simulink model "Bruening_4t_showshuffle"  (R2015a)
settings: Solver=ode4  SolverMode=MultiTasking  StartTime=0.0  StopTime=inf  FixedStep=BKIN_STEP_TIME  RelTol=1e-3
StartFcn:
  |  warndlg('Dexterit-E models cannot run under simulation. Please compile your model and run it from within Dexterit-E.');set_param(bdroot,'SimulationCommand','stop')
model workspace (MAT data in the model file):
  BKIN_STEP_TIME = 0.00025
  col_x = 1
  col_y = 2
  E_TARGET_ON = 3
  E_HOLD_AT_TARGET = 5
  LOGICAL_RADIUS = 4
  START_TARGET_COL = 1
  END_TARGET_COL = 2
  ROTATION_CENTER = 5
  WAIT_AT_1stTARGET_COL = 7
  MAXREACHTIME_COL = 8
  DELAY_POSTTRIAL_COL = 9
  E_STAY_CENTER = 2
  VISUAL_RADIUS = 3
  COLOR = 5
  ALTCOLOR = 6
  STROKECOLOUR = 7
  STROKEWIDTH = 9
  TARGET_EGG = 6
  LABEL_TEXT = 12
  LABEL_COLOUR = 13
  LABEL_HEIGHT = 14
  TEXT_DISPLAY_TARGET = 10
  ALTSTROKECOLOUR = 8
  SEGMENT_COUNT = 11
  E_TARGET_MISS = 6
  END_X = 10
  END_Y = 11
  E_LEFT_RING = 4
  E_START_BLOCK = 10
  BKIN_KINEMATIC_FRAME_SIZE = 400
  E_NO_EVENT = 1
  TARGET_IN_USE = 3
  R_PROB = 4
  E_R_TARG1 = 7
  E_M_TARG1 = 12
  E_R_TARG2 = 8
  E_M_TARG2 = 13
  E_R_TARG3 = 9
  E_M_TARG3 = 14
  E_R_TARG4 = 11
  E_M_TARG4 = 15
  WAIT_TIME = 12
  TONE_DURATION = 13
  FLASH_INTER = 14
  FLASH_NUM = 15
  BREAK_T1 = 16
  BREAK_T2 = 17
  ALTVISUAL_RADIUS = 15
  ALTCOLOR2 = 16
undefined symbols (not defined in the file or in its folder): slselsubs
libraries: Video x15, simulink x12, xpcrtudplib x12, xpcutilitieslib x10, xpcobsoletelib x8, ethercat x2, General x2, slrtlib x2, KINARM_general x1
(part 6 of 6)

== matlab function Bruening_4t_showshuffle/DataLogging/Poll KINARM/make KINData bus/splitKINData arm1 ==
  data: robot_row input; link_lengths output; pointer_offset output; shoulder_loc output; arm_orientation output; shoulder_ang output; elbow_ang output; shoulder_velocity output; elbow_velocity output; shoulder_acceleration output; elbow_acceleration output; joint_torque_cmd output; motor_torque_cmd output; link_angle output; link_velocity output; link_acceleration output; hand_position output; hand_velocity output; hand_acceleration output; motor_status output; force_sensor_force_uvw output; force_sensor_torque_uvw output; force_sensor_force_xyz output; force_sensor_torque_xyz output; force_sensor_timestamp output
function [link_lengths, pointer_offset, shoulder_loc, arm_orientation, ...
    shoulder_ang, elbow_ang, shoulder_velocity, elbow_velocity, shoulder_acceleration, elbow_acceleration, ...
    joint_torque_cmd, motor_torque_cmd, ...
    link_angle, link_velocity, link_acceleration, ...
    hand_position, hand_velocity, hand_acceleration, ...
    motor_status, ...
    force_sensor_force_uvw, force_sensor_torque_uvw, force_sensor_force_xyz, force_sensor_torque_xyz, force_sensor_timestamp] = splitKINData(robot_row)

link_lengths = robot_row(1,1:2);                % L1, L2 length in m
pointer_offset = robot_row(1,3);                % perpendicular distance from L2 to subject pointer (m)
shoulder_loc = robot_row(1,4:5);                % shoulder x,y position (m) (global coordinates)
arm_orientation = robot_row(1,6);                % subject's expected arm orientation (1: right, 2: left)
shoulder_ang = robot_row(1,7);				% shoulder joint angle, with correction for offsets (see above) (rad)
elbow_ang = robot_row(1,8);					% elbow joint angle, with correction for offsets (see above) (rad)
shoulder_velocity = robot_row(1,9);             % shoulder joint angular velocity (rad/s)
elbow_velocity = robot_row(1,10);               % elbow joint angular velocity (rad/s)
shoulder_acceleration = robot_row(1,11);        % shoulder joint angular acceleration (rad/s^2)
elbow_acceleration = robot_row(1,12);           % elbow joint angular acceleration (rad/s^2)
joint_torque_cmd = robot_row(1,13:14);          % commanded shoulder (1), and elbow (2) torque (Nm)
motor_torque_cmd = robot_row(1,15:16);          % commanded motor 1 (1) and 2 (2) torque (shoulder torque less elbow torque) (Nm)

link_angle = robot_row(1,17:18);                % upper arm angle with corrections, orientation-independent (see above) (rad)
link_velocity = robot_row(1,19:20);             % upper arm angular velocity, orientation-independent (see above) (rad/s)
link_acceleration = robot_row(1,21:22);         % upper arm angular acceleration, orientation-independent (see above) (rad/s^2)


hand_position = robot_row(1,23:24);             % fingertip position in x,y (m)
hand_velocity = robot_row(1,25:26);             % fingertip velocity in x,y (m/s)
hand_acceleration = robot_row(1,27:28);         % fingertip acceleration in x,y (m/s^2)

% shoulder_velocity_filt = robot_row(1,35);
% elbow_velocity_filt = robot_row(1,36);

motor_status = robot_row(1,37);                 % motor status (bitfield; each 0: motor enabled, 1: motor disabled/faulted)

force_sensor_force_uvw = robot_row(1,38:40);    % force measured by force sensor along u,v,w in its local coordinate system (N)
force_sensor_torque_uvw = robot_row(1,41:43);   % torque measured by force sensor along u,v,w in its local coordinate system (Nm)

force_sensor_force_xyz = robot_row(1,44:46);    % force measured by force sensor along x,y,z in the global coordinate system (N)
force_sensor_torque_xyz = robot_row(1,47:49);   % torque measured by force sensor along x in its local coordinate system (Nm)
force_sensor_timestamp = robot_row(1,50);       % The timestamp from the force sensor(s)

end

== matlab function Bruening_4t_showshuffle/DataLogging/Poll KINARM/make KINData bus/splitKINData arm2 ==
  data: robot_row input; link_lengths output; pointer_offset output; shoulder_loc output; arm_orientation output; shoulder_ang output; elbow_ang output; shoulder_velocity output; elbow_velocity output; shoulder_acceleration output; elbow_acceleration output; joint_torque_cmd output; motor_torque_cmd output; link_angle output; link_velocity output; link_acceleration output; hand_position output; hand_velocity output; hand_acceleration output; motor_status output; force_sensor_force_uvw output; force_sensor_torque_uvw output; force_sensor_force_xyz output; force_sensor_torque_xyz output; force_sensor_timestamp output
function [link_lengths, pointer_offset, shoulder_loc, arm_orientation, ...
    shoulder_ang, elbow_ang, shoulder_velocity, elbow_velocity, shoulder_acceleration, elbow_acceleration, ...
    joint_torque_cmd, motor_torque_cmd, ...
    link_angle, link_velocity, link_acceleration, ...
    hand_position, hand_velocity, hand_acceleration, ...
    motor_status, ...
    force_sensor_force_uvw, force_sensor_torque_uvw, force_sensor_force_xyz, force_sensor_torque_xyz, force_sensor_timestamp] = splitKINData(robot_row)

link_lengths = robot_row(1,1:2);                % L1, L2 length in m
pointer_offset = robot_row(1,3);                % perpendicular distance from L2 to subject pointer (m)
shoulder_loc = robot_row(1,4:5);                % shoulder x,y position (m) (global coordinates)
arm_orientation = robot_row(1,6);                % subject's expected arm orientation (1: right, 2: left)
shoulder_ang = robot_row(1,7);				% shoulder joint angle, with correction for offsets (see above) (rad)
elbow_ang = robot_row(1,8);					% elbow joint angle, with correction for offsets (see above) (rad)
shoulder_velocity = robot_row(1,9);             % shoulder joint angular velocity (rad/s)
elbow_velocity = robot_row(1,10);               % elbow joint angular velocity (rad/s)
shoulder_acceleration = robot_row(1,11);        % shoulder joint angular acceleration (rad/s^2)
elbow_acceleration = robot_row(1,12);           % elbow joint angular acceleration (rad/s^2)
joint_torque_cmd = robot_row(1,13:14);          % commanded shoulder (1), and elbow (2) torque (Nm)
motor_torque_cmd = robot_row(1,15:16);          % commanded motor 1 (1) and 2 (2) torque (shoulder torque less elbow torque) (Nm)

link_angle = robot_row(1,17:18);                % upper arm angle with corrections, orientation-independent (see above) (rad)
link_velocity = robot_row(1,19:20);             % upper arm angular velocity, orientation-independent (see above) (rad/s)
link_acceleration = robot_row(1,21:22);         % upper arm angular acceleration, orientation-independent (see above) (rad/s^2)


hand_position = robot_row(1,23:24);             % fingertip position in x,y (m)
hand_velocity = robot_row(1,25:26);             % fingertip velocity in x,y (m/s)
hand_acceleration = robot_row(1,27:28);         % fingertip acceleration in x,y (m/s^2)

% shoulder_velocity_filt = robot_row(1,35);
% elbow_velocity_filt = robot_row(1,36);
 
motor_status = robot_row(1,37);                 % motor status (bitfield; each 0: motor enabled, 1: motor disabled/faulted)

force_sensor_force_uvw = robot_row(1,38:40);    % force measured by force sensor along u,v,w in its local coordinate system (N)
force_sensor_torque_uvw = robot_row(1,41:43);   % torque measured by force sensor along u,v,w in its local coordinate system (Nm)

force_sensor_force_xyz = robot_row(1,44:46);    % force measured by force sensor along x,y,z in the global coordinate system (N)
force_sensor_torque_xyz = robot_row(1,47:49);   % torque measured by force sensor along x in its local coordinate system (Nm)
force_sensor_timestamp = robot_row(1,50);       % The timestamp from the force sensor(s)

end

== matlab function Bruening_4t_showshuffle/DataLogging/Poll KINARM/make KINData bus/splitKINDataGeneral ==
  data: kinarm_data input; active_arm output; delayEstimates output; servoCounter output; calibrationButtonBits output; handFF output; handFBArm output; handFBRadius output; handFBControl output; handFBColor output; hasGaze output; gazeFB output; gazeLocation output; gazeTimestamp output; gazePupilArea output; gazeEvent output
function [active_arm, delayEstimates, servoCounter, calibrationButtonBits, ...
    handFF, handFBArm, handFBRadius, handFBControl, handFBColor, hasGaze, gazeFB, ...
    gazeLocation, gazeTimestamp, gazePupilArea, gazeEvent] = splitKINData(kinarm_data)

    active_arm = kinarm_data(1);          % dominant KINARM for the experiment (1: arm 1, 2: arm 2)
    handFF = kinarm_data(2);              % duration of feed forward for position of hand feedback (s)
    handFBArm = kinarm_data(3);           % hand feedback arm (0: none, 1: dominant, 2: non-dominant, 3: both, 4: controlled by task program)
    handFBControl = kinarm_data(4);       % hand feedback settings source (0: GUI, 1: from task program)
    handFBColor = kinarm_data(5);         % feedback colour (RRRGGGBBB string converted to integer)
    handFBRadius = kinarm_data(6);        % feedback radius (m)

    delayEstimates = kinarm_data(8:11);   % primary encoders velocity(1), acceleration(2), seconadary enc velocity(3) and acceleration(4) delay estimate (s)
    servoCounter = kinarm_data(12);       % servo update count
    calibrationButtonBits = kinarm_data(13);  % EP calibration button status bitfield


    hasGaze = kinarm_data(14);            % is Gaze tracking hardware available
    gazeFB = kinarm_data(15);             % Gaze feedback (0: on, 1: controlled by task program)

    gazeLocation = kinarm_data(16:17);    % Gaze X,Y location in global coordinates
    gazeTimestamp = kinarm_data(18);      % Gaze Timestamp in seconds
    gazePupilArea = kinarm_data(19);      % Gaze pupil area
    gazeEvent = kinarm_data(20:22);       % Gaze Event ID(1), start time(2), end time (3) 
end

== matlab function Bruening_4t_showshuffle/DataLogging/Poll KINARM/split_primary/split_primary ==
  data: primary_data input; link_angles output; link_velocities output; link_acceleration output
function [link_angles, link_velocities, link_acceleration] = splitPrimary(primary_data)
   link_angles = primary_data(1:2);
   link_velocities = primary_data(3:4);
   link_acceleration = primary_data(5:6);
end

== matlab function Bruening_4t_showshuffle/DataLogging/Poll KINARM/split_primary/split_primary1 ==
  data: primary_data input; link_angles output; link_velocities output; link_acceleration output
function [link_angles, link_velocities, link_acceleration] = splitPrimary(primary_data)
   link_angles = primary_data(1:2);
   link_velocities = primary_data(3:4);
   link_acceleration = primary_data(5:6);
end

== matlab function Bruening_4t_showshuffle/DataLogging/Receive_Gaze/Create timestamp ==
  data: time_in input; timestamp_out output; start_time_out output
function [timestamp_out, start_time_out] = fcn(time_in)

persistent start_time
persistent last_time

if isempty(start_time)
   start_time = -1;
end

if isempty(last_time)
    last_time = -1;
end

if start_time == -1 && time_in ~= 0
    start_time = time_in;
end

%if the clock has flipped over then in order to get the time
%right this will add the time before the flip to the current time.
if time_in < start_time
    start_time = -(last_time - start_time);
end

timestamp_out = (time_in - start_time) / 1000.0;
last_time = time_in;
start_time_out = start_time;

== matlab function Bruening_4t_showshuffle/DataLogging/Receive_Gaze/Embedded MATLAB Function1 ==
  data: input input; pupil_area_PIXELS input; tracking_status input; tracking_available input; camtheta input; camera_GLOBAL input; focal_length input; gazeXYCalculated output; target_distance_in input; pupil_area_GLOBAL output
function [gazeXYCalculated, pupil_area_GLOBAL] = fcn(input, pupil_area_PIXELS, tracking_status, tracking_available, camtheta,camera_GLOBAL, focal_length, target_distance_in)

% The following are some details on the Eyelink camera
EL_target_distance_scaling_factor = 10000;					%target distance is reported by Eyelink in 1/10 of mm units
EL_pix_per_mm = 200;										%there are 200 pixels/mm on the Eyelink 1000 camera sensor

raw_pupil = [input(1) input(2)];
href = [input(3); input(4); 0];
target_distance = target_distance_in / EL_target_distance_scaling_factor;		% distance of the target from the camera (m)

%if there is a blink or other problem then send out errors. C3D file does not like NaN, so we output -100.
if tracking_status == 4 || tracking_available == 0 || (href(1) == 0 && href(2) == 0) || (raw_pupil(1) == -32768 && raw_pupil(2) == -32768)
    gazeXYCalculated = [-100; -100];
	pupil_area_GLOBAL = -100;
% % % 	testing = [0 0 0 0 0 0];
% % % 	testing2 = [0; 0; 0; 0; 0; 0];
    return
end

[Rx Ry Rz] = calc_R_from_angles(camtheta(1), camtheta(2), 0);
R_CMRA2GLBL = Rx * Ry;
%R_GLBL2CMRA = R_CMRA2GLBL';

%camera_GLOBAL_Trans = camera_GLOBAL';
pupil_XY_Sensor = convertPupilToSensor(raw_pupil(1), raw_pupil(2), EL_pix_per_mm);
[gaze_GLOBAL, pupil_GLOBAL] = calc_GAZE(pupil_XY_Sensor, target_distance, href, focal_length, camera_GLOBAL, R_CMRA2GLBL);
gazeXYCalculated = gaze_GLOBAL(1:2);

%%convert the pupil area from pixels on the sensor, to m^2, correcting for camera and gaze angle
% pupil area on the camera sensor, in m^2
pupil_area_SENSOR = pupil_area_PIXELS / ( (EL_pix_per_mm * 1000 ) ^ 2);		

% pupil area in the global workspace, projected onto a plane parallel to the camera sensor in m^2
pupil_area_GLOBAL_projection = pupil_area_SENSOR * (target_distance / focal_length) ^ 2; 

% create a unit vector that is normal to the camera sensor, in GLOBAL coordinates
sensor_unit_vector_GLOBAL = R_CMRA2GLBL * [0; 0; 1];

% create a unit vector for the subject's gaze
gaze_vector_GLOBAL = pupil_GLOBAL - gaze_GLOBAL;
gaze_unit_vector_GLOBAL = gaze_vector_GLOBAL / norm(gaze_vector_GLOBAL);

% calculate the cosine of the angle between the unit vectors for gaze and the camera sensor
cos_gaze_camera_angle = dot(sensor_unit_vector_GLOBAL, gaze_unit_vector_GLOBAL); 

% correct the pupil area to account for the angle of the eye relative to the camera sensor plane
% We assume that the pupil is circular. In the plane formed by the two vectors, the distance needs 
% to be scaled by cos(theta). In the perpendicular plane, there is no scaling. Hence we do NOT 
% square the cos(theta) and the area is only corrected for by 1 / cos(theta). 
pupil_area_GLOBAL = pupil_area_GLOBAL_projection / cos_gaze_camera_angle;

% % % % For testing
% % % gaze_camera_angle  = acos(cos_gaze_camera_angle) * 180/pi();
% % % HREF_angle = atan2( norm(href), 15000) * 180 / pi();
% % % testing = [pupil_area_SENSOR*1e6, pupil_area_GLOBAL_projection*1e6, pupil_area_GLOBAL*1e6, gaze_camera_angle, HREF_angle, cos_gaze_camera_angle];
% % % testing2 = [sensor_unit_vector_GLOBAL; gaze_unit_vector_GLOBAL];



%% Functions
function [gaze_est_GLOBAL, pupil_GLOBAL] = calc_GAZE(pupil_SENSOR, target_distance, HREF_HREF, focal_length, camera_GLOBAL, R_CMRA2GLBL)
    % This function estimates GAZE based on data from the Eyelink.  To be used
    % during 'running' of a task. 

    % Convert pupil location from Eyelink sensor frame to camera reference
    % frame with camera at origin and rotated to camera's angle (W-axis along
    % camera's point of view)  
    pupil_CAMERA = [pupil_SENSOR * target_distance / focal_length; target_distance];
    pupil_distance = norm(pupil_CAMERA);

    % Rotation matrix to convert from HREF coordinates to camera coordinates.
    % HREF z-axis is defined as ray from camera to pupil.
    R_HREF2CMRA = calc_R_from_vectors(pupil_CAMERA, [0; 0; 1]);

    % Convert the HREF from HREF coordinates to canera coordinates.  Scale,
    % then rotate. 
    HREF_CAMERA = R_HREF2CMRA * (HREF_HREF * pupil_distance / 15000);

    % Then convert pupil and HREF locations from camera frame to global frame
    % by rotating and then shifting origins. 
    pupil_GLOBAL = R_CMRA2GLBL * pupil_CAMERA + camera_GLOBAL';
    HREF_GLOBAL = R_CMRA2GLBL * HREF_CAMERA + camera_GLOBAL';

    % Find intersection of gaze_ray (from pupil to HREF) with the subject_display plane
    norm_vector = [0; 0; 1];		% In the KINARM VR setup, the Z-axis is defined as normal to the subject display
    point_on_plane = [0; 0; 0];		% In the KINARM VR setup, the origin is defined as on the subject display plane

    % display([pupil_GLOBAL HREF_GLOBAL])
    gaze_est_GLOBAL = plane_line_intersect(norm_vector, point_on_plane, pupil_GLOBAL, HREF_GLOBAL);

function pupil_XY_Sensor = convertPupilToSensor(pupilX, pupilY, pix_per_mm)
%         Returns the projection of the pupil on the camera sensor in meters, based on inputs in some raw unit (not pixels)

    % the following constants are from Jiye, email Nov 7, 2011
    LEFTDROP = 32;				%pixels dropped at left of sensor
    TOPDROP = 48;				%lines dropped at top of sensor
    const_x = 7*176;			%no idea what this is.  Maybe number of pixels???
    const_y = 4*184 + 188;		%no idea what this is.  Maybe number of pixels???

    % from Jiye. Not sure excatly what they are (probably camera center in pixels)
    cam_rot_cx = const_x / 2 + LEFTDROP;			
    cam_rot_cy = const_y / 2 +TOPDROP;

    hor = 30000;
    lor = -30000;
    hr = 0.9;
    lr = 0.1;
    ld = 50;
    hdx = 1200;		%hmmm almost same as const_x, which is 1232
    hdy = 920;		%hmmm almost same as const_y, which is 924

    scx = (hor-lor) / (hdx - ld) / (hr-lr);
    ofx = lor - (ld + (hdx - ld) * lr )* scx;

    scy = (hor-lor) / (hdy - ld) / (hr-lr);
    ofy = lor - (ld + (hdy - ld) * lr )* scy;

    % calculate the pupil in camera sensor coordinates (pixels)
    px = (pupilX - ofx) / scx;
    py = (pupilY - ofy) / scy;

    ppl_mmX = - ( (cam_rot_cx - px) / pix_per_mm );
    ppl_mmY =   ( (cam_rot_cy - py) / pix_per_mm );

    pupil_XY_Sensor = [ppl_mmX / 1000; ppl_mmY / 1000];
    
function [Rx Ry Rz] = calc_R_from_angles(xrot, yrot, zrot)
    % This function creates the three rotation matrices for rotations about the
    % x, y and z axes.  Input rotations are in degrees.

    xrot = xrot/180*pi;		%convert to radians
    yrot = yrot/180*pi;		%convert to radians
    zrot = zrot/180*pi;		%convert to radians
    Rx = [1 0 0; 0 cos(xrot) -sin(xrot); 0 sin(xrot) cos(xrot)]; 
    Ry = [cos(yrot) 0 sin(yrot); 0 1 0; -sin(yrot) 0 cos(yrot)]; 
    Rz = [cos(zrot) -sin(zrot) 0; sin(zrot) cos(zrot) 0 ; 0 0 1]; 

    
function R = calc_R_from_vectors(v1, v2)
    % This function calculates a rotation matrix, given two vectors, such that
    % the rotation matrix will rotate from v1 to v2.

    rot_axis = cross(v2, v1);			%axis that is perpendicular to the two vectors

    % If either of the vectors v1 or v2 is = [0 0 0], or if they are parallel
    % (i.e. norm(rot_axis) == 0), then there is no rotation.  But math errors
    % will occur, so we need to check for these cases.   
    if (norm(v1) == 0) || (norm(v2) == 0)	|| (norm(rot_axis) == 0)
        R = eye(3);																%identity matrix results in no rotation
    else
        rot_angle = asin( norm(rot_axis) / norm(v1) / norm(v2) );				%angle of rotation about rot_axis
        n = rot_axis / norm(rot_axis);											%normalize to get a unit vector for the rotation
        n_cross_product_matrix = [ 0 -n(3) n(2); n(3) 0 -n(1); -n(2) n(1) 0];	%def'n of cross product matrix
        cosA = cos(rot_angle);
        sinA = sin(rot_angle);
        R = eye(3) * cosA + sinA * n_cross_product_matrix + (1 - cosA) * (n * n');
    % 	display(rot_angle);
    end


function I = plane_line_intersect(n,V0,P0,P1)
    %plane_line_intersect computes the intersection of a plane and a segment(or
    %a straight line)
    % Inputs: 
    %       n: normal vector of the Plane 
    %       V0: any point that belongs to the Plane 
    %       P0: end point 1 of the segment P0P1
    %       P1:  end point 2 of the segment P0P1
    %
    %Outputs:
    %      I    is the point of interection 
    %     Check is (DELETED AND NOT USED HERE) an indicator:
    %      0 => disjoint (no intersection)
    %      1 => the plane intersects P0P1 in the unique point I
    %      2 => the segment lies in the plane
    %      3=>the intersection lies outside the segment P0P1
    %
    % Example:
    % Determine the intersection of following the plane x+y+z+3=0 with the segment P0P1:
    % The plane is represented by the normal vector n=[1 1 1]
    % and an arbitrary point that lies on the plane, ex: V0=[1 1 -5]
    % The segment is represented by the following two points
    % P0=[-5 1 -1]
    %P1=[1 2 3]   
    % [I,check]=plane_line_intersect([1 1 1],[1 1 -5],[-5 1 -1],[1 2 3]);

    %This function is written by :
    %                             Nassim Khaled
    %                             Wayne State University
    %                             Research Assistant and Phd candidate
    %If you have any comments or face any problems, please feel free to leave
    %your comments and i will try to reply to you as fast as possible.

    I=[0; 0; 0];
    u = P1-P0;
    w = P0 - V0;
    D = dot(n,u);
    N = -dot(n,w);
    check=0;
    if abs(D) < 10^-7        % The segment is parallel to plane
            if N == 0           % The segment lies in plane
                check=2;
                return
            else
                check=0;       %no intersection
                return
            end
    end

    %compute the intersection parameter
    sI = N / D;
    I = P0+ sI.*u;

== matlab function Bruening_4t_showshuffle/DataLogging/Receive_Gaze/clean_packet ==
  data: pack_in input; pack_out output; len_out output; len_in input
function [pack_out, len_out] = clean_packet(pack_in, len_in)

%for some reason, during calibration we can get very large packets that 
%blow up the c code for parsing the packets. If we get a large packet
%we can ignore it.

if len_in < 512
    pack_out = pack_in;
    len_out = len_in;
else
    pack_out = zeros(512, 1, 'uint8');
    len_out = int32(0);
end

== matlab function Bruening_4t_showshuffle/DataLogging/Receive_Gaze/convert to seconds ==
  data: event_data input; event_data_out output; start_time input; eyelink_timestamp input
function event_data_out = fcn(event_data, start_time, eyelink_timestamp)

persistent last_timestamp

if isempty(last_timestamp)
	last_timestamp = uint32(0);
end

%DEX-3313 if eyelink has stopped sending us data then we should not flood
%Dex with events.
if last_timestamp == eyelink_timestamp
	event_data_out = [0; 0; 0];
	return
end

last_timestamp = eyelink_timestamp;
event_data_out = event_data;

if event_data(1) ~= 0
    event_data_out(2) = (event_data(2) - start_time) / 1000.0;
    event_data_out(3) = (event_data(3) - start_time) / 1000.0;
end

== matlab function Bruening_4t_showshuffle/DataLogging/compare encoders/delta ==
  data: secondaryEncAngles input; deltas output; primaryEncAngles input
function deltas = fcn(secondaryEncAngles, primaryEncAngles)
%#eml

deltas = secondaryEncAngles - primaryEncAngles;

== matlab function Bruening_4t_showshuffle/displayBlockLabel ==
  data: VCODE input; VCODE_out output; blocknum input
function VCODE_out  = displayBlockLabel(VCODE, blocknum)
%#codegen
blocknum = double(blocknum);
text_prefix = 'New Block';
endPrefix = 14 + length(text_prefix);
VCODE(15:endPrefix) = uint8(text_prefix);

max_block = 1000;
if blocknum >= max_block
    blocknum = 9.99999 * max_block;
end
power_vals = nan(1,3);
power10 = floor(log10(blocknum));
if blocknum == 0
    power10 = 0;
end
for i = 0:power10
    power_vals(i+1) = power10-i;
end

power_vals = power_vals(~isnan(power_vals));

% for p = 1:length(power_vals);
    %VCODE(endPrefix+p) = getChar(blocknum,10^(power_vals(p)));
% end

VCODE(endPrefix+1) = 0; %terminate the new string
VCODE_out = VCODE;
end


function cc = getChar(number, dec)
%in simulink there is no nice way to convert a number to s string
%so what we are doing here is converting a single digit to a character.
%48 is ascii for '0', so this gets the least significant digit before
%the decimal and converts to ascii.
cc = floor(mod(number / dec, 10)) + 48;
end

== matlab function Bruening_4t_showshuffle/displayRestTag ==
  data: VCODE input; VCODE_out output
function VCODE_out  = displayRestTag(VCODE)
%#codegen
text_prefix = 'Take a Break';
endPrefix = 14 + length(text_prefix);
VCODE(15:endPrefix) = uint8(text_prefix);
VCODE_out = VCODE;
end

== matlab function Bruening_4t_showshuffle/displayScoreTrialL1 ==
  data: VCODE input; VCODE_out output; score_ret input
function VCODE_out  = displayScoreTrialL1(VCODE, score_ret)
%#codegen

text_prefix = 'WOW! ';
endPrefix = 14 + length(text_prefix);
VCODE(15) = 87;  %'W'
VCODE(16) = 79;  %'O'
VCODE(17) = 87;
VCODE(18) = 33;  %'!'
VCODE(19) = 32;  %' ' space

max_scoreP = 10^5;
if score_ret >= max_scoreP
    score_ret = 9.99999 * max_scoreP;
end
power_vals = nan(1,5);
power10 = floor(log10(score_ret));
if score_ret == 0
    power10 = 0;
end
for i = 0:power10
    power_vals(i+1) = power10-i;
end

power_vals = power_vals(~isnan(power_vals));

for p = 1:length(power_vals);
    VCODE(endPrefix+p) = getChar(score_ret,10^(power_vals(p)));
end

VCODE(endPrefix+length(power_vals)+1) = 0; %terminate the new string
VCODE_out = VCODE;
end


function cc = getChar(number, dec)
%in simulink there is no nice way to convert a number to s string
%so what we are doing here is converting a single digit to a character.
%48 is ascii for '0', so this gets the least significant digit before
%the decimal and converts to ascii.
cc = floor(mod(number / dec, 10)) + 48;
end

== stateflow chart Bruening_4t_showshuffle/DataLogging/Poll KINARM/control read write ==
  settings: sampleTime=0.0005
  state RunSim/
    during:
    simulation;
    buildKINData
  state RunECat/
    during:
    ecat;
    buildKINData;
  state RunPMAC/
    during:
    pmac;
    buildKINData;
  (default) -> (junction 216)
  (junction 216) -> RunSim [order 3]
  (junction 216) -> RunPMAC [order 2] : [system_type == 1]
  (junction 216) -> RunECat [order 1] : [system_type == 2]
  data: system_type input double
  events: simulation output FUNCTION_CALL_EVENT; ecat output FUNCTION_CALL_EVENT; pmac output FUNCTION_CALL_EVENT; buildKINData output FUNCTION_CALL_EVENT

== matlab function Bruening_4t_showshuffle/displayMissTarg ==
  data: VCODE input; VCODE_out output
function VCODE_out  = displayMissTarg(VCODE)
%#codegen
text_prefix = 'Aim for the Target!';
endPrefix = 14 + length(text_prefix);
VCODE(15:endPrefix) = uint8(text_prefix);
VCODE(endPrefix+1) = 0; %terminate the new string
VCODE_out = VCODE;
end
